simulink model "Rail_SetPoint"  (R2016b)
settings: configuration reference "CodeGenConfigSet" (kept outside this file)
values from neighbouring files (symbols this model uses):
  Rail_dpSetPointDec_CUR = Calibration.Parameter    [init_Rail_SetPoint.m]    (also in init_Rail_SetPoint_SIL.m = Simulink.Parameter)
  Rail_dpSetPointDec_CURX = Calibration.Parameter    [init_Rail_SetPoint.m]    (also in init_Rail_SetPoint_SIL.m = Simulink.Parameter)
  Rail_dpSetPointDec_MAP = Calibration.Parameter    [init_Rail_SetPoint.m]    (also in init_Rail_SetPoint_SIL.m = Simulink.Parameter)
  Rail_dpSetPointDec_MAPX = Calibration.Parameter    [init_Rail_SetPoint.m]    (also in init_Rail_SetPoint_SIL.m = Simulink.Parameter)
  Rail_dpSetPointDec_MAPY = Calibration.Parameter    [init_Rail_SetPoint.m]    (also in init_Rail_SetPoint_SIL.m = Simulink.Parameter)
  Rail_dpSetPointInc_MAP = Calibration.Parameter    [init_Rail_SetPoint.m]    (also in init_Rail_SetPoint_SIL.m = Simulink.Parameter)
  Rail_dpSetPointInc_MAPX = Calibration.Parameter    [init_Rail_SetPoint.m]    (also in init_Rail_SetPoint_SIL.m = Simulink.Parameter)
  Rail_dpSetPointInc_MAPY = Calibration.Parameter    [init_Rail_SetPoint.m]    (also in init_Rail_SetPoint_SIL.m = Simulink.Parameter)
  Rail_dpSetPointIncLim_MAP = Calibration.Parameter    [init_Rail_SetPoint.m]    (also in init_Rail_SetPoint_SIL.m = Simulink.Parameter)
  Rail_dpSetPointIncLim_MAPX = Calibration.Parameter    [init_Rail_SetPoint.m]    (also in init_Rail_SetPoint_SIL.m = Simulink.Parameter)
  Rail_dpSetPointIncLim_MAPY = Calibration.Parameter    [init_Rail_SetPoint.m]    (also in init_Rail_SetPoint_SIL.m = Simulink.Parameter)
  Rail_pEnvpSetPointIncHi_C = Calibration.Parameter    [init_Rail_SetPoint.m]    (also in init_Rail_SetPoint_SIL.m = Simulink.Parameter)
  Rail_pEnvpSetPointIncLo_C = Calibration.Parameter    [init_Rail_SetPoint.m]    (also in init_Rail_SetPoint_SIL.m = Simulink.Parameter)
  Rail_pSetPointBasEOM0_MAP = Calibration.Parameter    [init_Rail_SetPoint.m]    (also in init_Rail_SetPoint_SIL.m = Simulink.Parameter)
  Rail_pSetPointBasEOM0_MAPX = Calibration.Parameter    [init_Rail_SetPoint.m]    (also in init_Rail_SetPoint_SIL.m = Simulink.Parameter)
  Rail_pSetPointBasEOM0_MAPY = Calibration.Parameter    [init_Rail_SetPoint.m]    (also in init_Rail_SetPoint_SIL.m = Simulink.Parameter)
  Rail_pSetPointErrLoLim_CUR = Calibration.Parameter    [init_Rail_SetPoint.m]    (also in init_Rail_SetPoint_SIL.m = Simulink.Parameter)
  Rail_pSetPointErrLoLim_CURX = Calibration.Parameter    [init_Rail_SetPoint.m]    (also in init_Rail_SetPoint_SIL.m = Simulink.Parameter)
  Rail_pSetPointLimNFlTemp_MAP = Calibration.Parameter    [init_Rail_SetPoint.m]    (also in init_Rail_SetPoint_SIL.m = Simulink.Parameter)
  Rail_pSetPointLimNFlTemp_MAPX = Calibration.Parameter    [init_Rail_SetPoint.m]    (also in init_Rail_SetPoint_SIL.m = Simulink.Parameter)
  Rail_pSetPointLimNFlTemp_MAPY = Calibration.Parameter    [init_Rail_SetPoint.m]    (also in init_Rail_SetPoint_SIL.m = Simulink.Parameter)
  Rail_pSetPointRed_C = Calibration.Parameter    [init_Rail_SetPoint.m]    (also in init_Rail_SetPoint_SIL.m = Simulink.Parameter)
  Rail_swtDynLim_C = Calibration.Parameter    [init_Rail_SetPoint.m]    (also in init_Rail_SetPoint_SIL.m = Simulink.Parameter)
  Rail_swtIncLim_C = Calibration.Parameter    [init_Rail_SetPoint.m]    (also in init_Rail_SetPoint_SIL.m = Simulink.Parameter)
  Rail_swtPSetPointSrc_C = Calibration.Parameter    [init_Rail_SetPoint.m]    (also in init_Rail_SetPoint_SIL.m = Simulink.Parameter)
  Rail_swtqIncSel_C = Calibration.Parameter    [init_Rail_SetPoint.m]    (also in init_Rail_SetPoint_SIL.m = Simulink.Parameter)
  Rail_swtStatLim_C = Calibration.Parameter    [init_Rail_SetPoint.m]    (also in init_Rail_SetPoint_SIL.m = Simulink.Parameter)
  SigTst_pSetPoint_C = Calibration.Parameter    [init_Rail_SetPoint.m]    (also in init_Rail_SetPoint_SIL.m = Simulink.Parameter)
  SigTst_swtSetPoint_C = Calibration.Parameter    [init_Rail_SetPoint.m]    (also in init_Rail_SetPoint_SIL.m = Simulink.Parameter)
undefined symbols (not defined in the file or in its folder): EngState_conv, Rail_SetPoint_DT, RailCtl_State_conv, Switch_conv
libraries: CXLib x5
settings Model: Creator=lenovo  LastModifiedBy=dulinggang
settings ConfigSetRef: SourceLocation=Base Workspace

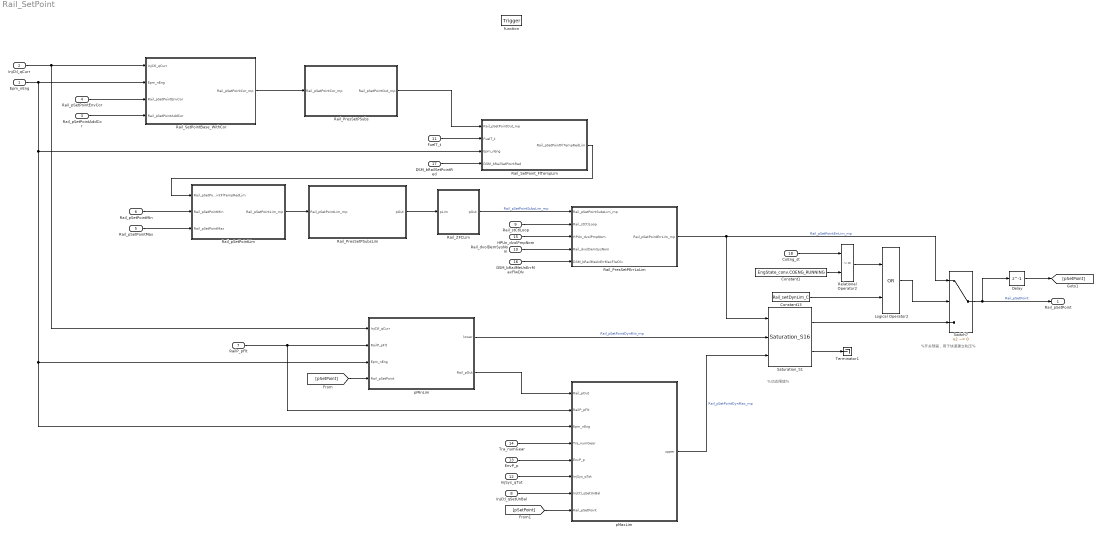
== system Rail_SetPoint ==
  note: %动态限值%
  note: %开关预留，用于快速建立轨压%
  Epm_nEng : Inport  Tag=rpm  Description=Engine speed  OutMin=0  OutMax=6000  OutDataTypeStr=EngSpeed_rpm
  InjCtl_qCurr : Inport  Tag=mg/hub  Description=Torque generating engine fuel injection quantity  Port=2  OutMin=-319  OutMax=319  OutDataTypeStr=FuelMass_mg_hub
  Rail_pSetPointAddCor : Inport  Tag=bar  Description=Buffer variable for additional correction rail setpoint values which were received via the remote function Rail_SetPointAddCor.  Port=3  OutMin=-2500  OutMax=2500  OutDataTypeStr=RailPressure_bar
  Rail_pSetPointEnvCor : Inport  Tag=bar  Description=Corrected rail pressure setpoint based on environmental conditions (for present operation mode)  Port=4  OutMin=-2500  OutMax=2500  OutDataTypeStr=RailPressure_bar
  Rail_pSetPointMax : Inport  Tag=bar  Description=Maximum rail pressure setpoint  Port=5  OutMin=-2500  OutMax=2500  OutDataTypeStr=RailPressure_bar
  Rail_pSetPointMin : Inport  Tag=bar  Description=Minimum rail pressure setpoint  Port=6  OutMin=-2500  OutMax=2500  OutDataTypeStr=RailPressure_bar
  RailP_pFlt : Inport  Tag=bar  Description=Maximum rail pressure of the last 10 sampling cycle  Port=7  OutMin=0  OutMax=2500  OutDataTypeStr=RailPressure_bar
  InjCtl_qSetUnBal : Inport  Tag=mg/hub  Description=Current injection quantity  Port=8  OutMin=-319  OutMax=319  OutDataTypeStr=FuelMass_mg_hub
  Rail_stCtlLoop : Inport  Description=State of the rail pressure governor control  Port=9  OutDataTypeStr=Enum: RailCtl_State_conv
  Rail_dvolDemSysNom : Inport  Tag=mm^3/s  Description=Volume flow demanded overall for a nominal injection system  Port=10  OutMin=-327680  OutMax=327670  OutDataTypeStr=FuelVol_mm3_s
  FuelT_t : Inport  Tag=deg  Description=Temperature of fuel  Port=11  OutMin=-50  OutMax=150  OutDataTypeStr=Temp_deg
  InjSys_qTot : Inport  Tag=mg/hub  Description=Total engine injection quantity  Port=12  OutMin=-319  OutMax=319  OutDataTypeStr=FuelMass_mg_hub
  EnvP_p : Inport  Tag=kPa  Description=Barometric pressure  Port=13  OutMin=0  OutMax=3276  OutDataTypeStr=AirPressure_kPa
  Tra_numGear : Inport  Description=Current gear information  Port=14  OutMin=-128  OutMax=127  OutDataTypeStr=Tra_num
  HPUn_dvolPmpNom : Inport  Tag=mm^3/s  Description=Pump Nominal value  Port=15  OutMin=0  OutMax=50000  OutDataTypeStr=FuelVol_mm3_s
  DSM_bRailMeUnErrMaxFlwDlv : Inport  Description=state of Fid_RailMeUnErrMaxFlwDlv  Port=16  OutMin=0  OutMax=1  OutDataTypeStr=boolean
  DSM_bRailSetPointRed : Inport  Description=state of FId_RailSetPointRed  Port=17  OutMin=0  OutMax=1  OutDataTypeStr=boolean
  CoEng_st : Inport  Description=Engine coordinator state  Port=18  OutDataTypeStr=Enum: EngState_conv
  function : TriggerPort  TriggerType=function-call  VariantControl=Variant
  Constant1 : Constant  Value=EngState_conv.COENG_RUNNING
  Constant13 : Constant  Value=Rail_swtDynLim_C
  Delay : Delay  DelayLength=1  InitialCondition=0
  Logical Operator2 : Logic  Operator=OR  AllPortsSameDT=off  OutDataTypeStr=boolean
  Rail_PresSetPErrLoLim : Subsystem
  Rail_PresSetPSubs : Subsystem
  Rail_PresSetPSubsLim : Subsystem
  Rail_SetPointBase_WithCor : Subsystem
  Rail_SetPoint_FlTempLim : Subsystem
  Rail_ZFCLim : Subsystem
  Rail_pSetPointLim : Subsystem
  Relational Operator2 : RelationalOperator  Operator=~=  OutDataTypeStr=boolean  RndMeth=Simplest  InputSameDT=on
  Saturation_S1 : CXLib/Saturation_S16  RequirementInfo={'other' 'Rail_requirements.doc' '@Simulink_requirement_item_42' 'true' '目标轨压动态限值' '' } %GIDa_002271f1_d5a1_4f79_991c_8acc6585766a
  Switch7 : Switch  Criteria=u2 ~= 0  InputSameDT=on
  Terminator1 : Terminator
  pMaxLim : Subsystem
  pMinLim : Subsystem
  Rail_pSetPoint : Outport  Tag=bar  Description=Rail pressure setpoint  OutMin=-2500  OutMax=2500  OutDataTypeStr=RailPressure_bar
  wires:
  Saturation_S1/1 -> Switch7/3
  Rail_SetPointBase_WithCor/1(Rail_pSetPointCor_mp) -> Rail_PresSetPSubs/1(Rail_pSetPointCor_mp)
  Rail_stCtlLoop/1 -> Rail_PresSetPErrLoLim/2(Rail_stCtlLoop)
  Rail_dvolDemSysNom/1 -> Rail_PresSetPErrLoLim/4(Rail_dvolDemSysNom)
  HPUn_dvolPmpNom/1 -> Rail_PresSetPErrLoLim/3(HPUn_dvolPmpNom)
  Delay/1 -> [pSetPoint]
  Switch7/1 -> Rail_pSetPoint/1, Delay/1  "Rail_pSetPoint"
  RailP_pFlt/1 -> pMinLim/2(RailP_pFlt), pMaxLim/2(RailP_pFlt)
  Saturation_S1/2 -> Terminator1/1
  Rail_PresSetPErrLoLim/1(Rail_pSetPointErrLim_mp) -> Switch7/1, Saturation_S1/1  "Rail_pSetPointErrLim_mp"
  Rail_ZFCLim/1(pOut) -> Rail_PresSetPErrLoLim/1(Rail_pSetPointSubsLim_mp)  "Rail_pSetPointSubsLim_mp"
  Rail_PresSetPSubsLim/1(pOut) -> Rail_ZFCLim/1(pLim)
  Rail_pSetPointEnvCor/1 -> Rail_SetPointBase_WithCor/3(Rail_pSetPointEnvCor)
  Rail_pSetPointAddCor/1 -> Rail_SetPointBase_WithCor/4(Rail_pSetPointAddCor)
  Epm_nEng/1 -> pMaxLim/3(Epm_nEng), pMinLim/3(Epm_nEng), Rail_SetPoint_FlTempLim/3(Epm_nEng), Rail_SetPointBase_WithCor/2(Epm_nEng)
  InjCtl_qCurr/1 -> pMinLim/1(InjCtl_qCurr), Rail_SetPointBase_WithCor/1(InjCtl_qCurr)
  DSM_bRailMeUnErrMaxFlwDlv/1 -> Rail_PresSetPErrLoLim/5(DSM_bRailMeUnErrMaxFlwDlv)
  Rail_PresSetPSubs/1(Rail_pSetPointOut_mp) -> Rail_SetPoint_FlTempLim/1(Rail_pSetPointOut_mp)
  FuelT_t/1 -> Rail_SetPoint_FlTempLim/2(FuelT_t)
  DSM_bRailSetPointRed/1 -> Rail_SetPoint_FlTempLim/4(DSM_bRailSetPointRed)
  Rail_SetPoint_FlTempLim/1(Rail_pSetPointFlTempRedLim) -> Rail_pSetPointLim/1(Rail_pSetPointFlTempRedLim)
  Rail_pSetPointMin/1 -> Rail_pSetPointLim/2(Rail_pSetPointMin)
  Rail_pSetPointMax/1 -> Rail_pSetPointLim/3(Rail_pSetPointMax)
  Rail_pSetPointLim/1(Rail_pSetPointLim_mp) -> Rail_PresSetPSubsLim/1(Rail_pSetPointLim_mp)
  pMinLim/1(lower) -> Saturation_S1/2  "Rail_pSetPointDynMin_mp"
  pMinLim/2(Rail_pOut) -> pMaxLim/1(Rail_pOut)
  Tra_numGear/1 -> pMaxLim/4(Tra_numGear)
  EnvP_p/1 -> pMaxLim/5(EnvP_p)
  InjSys_qTot/1 -> pMaxLim/6(InjSys_qTot)
  InjCtl_qSetUnBal/1 -> pMaxLim/7(InjCtl_qSetUnBal)
  pMaxLim/1(upper) -> Saturation_S1/3  "Rail_pSetPointDynMax_mp"
  [pSetPoint] -> pMinLim/4(Rail_pSetPoint)
  [pSetPoint] -> pMaxLim/8(Rail_pSetPoint)
  CoEng_st/1 -> Relational Operator2/1
  Constant1/1 -> Relational Operator2/2
  Relational Operator2/1 -> Logical Operator2/1
  Constant13/1 -> Logical Operator2/2
  Logical Operator2/1 -> Switch7/2

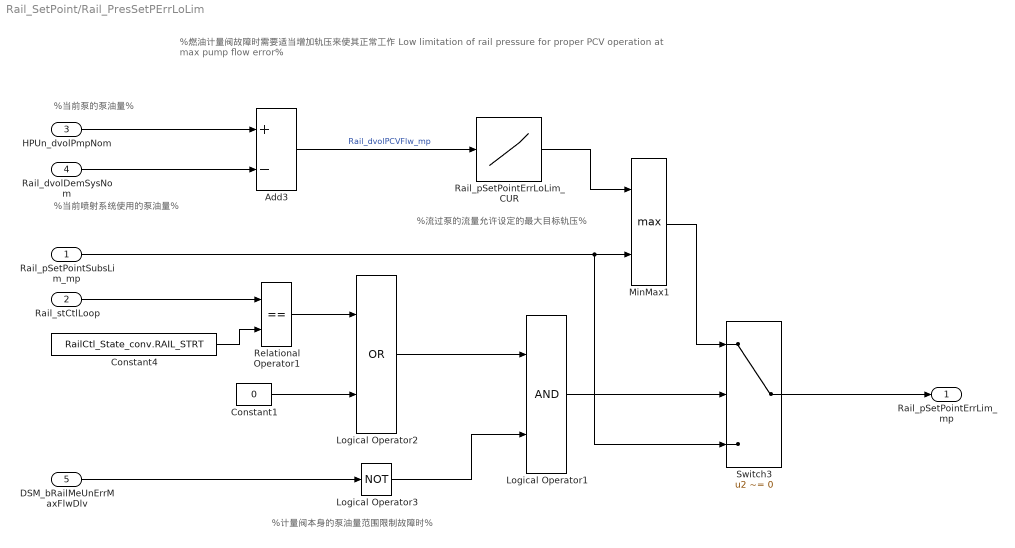
== system Rail_SetPoint/Rail_PresSetPErrLoLim ==
  note: %燃油计量阀故障时需要适当增加轨压来使其正常工作
      | Low limitation of rail pressure for proper PCV operation at max pump ﬂow error%
  note: %当前泵的泵油量%
  note: %当前喷射系统使用的泵油量%
  note: %流过泵的流量允许设定的最大目标轨压%
  note: %计量阀本身的泵油量范围限制故障时%
  Rail_pSetPointSubsLim_mp : Inport
  Rail_stCtlLoop : Inport  Port=2
  HPUn_dvolPmpNom : Inport  Port=3
  Rail_dvolDemSysNom : Inport  Port=4
  DSM_bRailMeUnErrMaxFlwDlv : Inport  Description=state of Fid_RailMeUnErrMaxFlwDlv  Port=5  OutMin=0  OutMax=1  OutDataTypeStr=boolean
  Add3 : Sum  Inputs=+-  OutDataTypeStr=Inherit: Inherit via back propagation  InputSameDT=on
  Constant1 : Constant  Value=0  OutDataTypeStr=Inherit: Inherit via back propagation
  Constant4 : Constant  Value=RailCtl_State_conv.RAIL_STRT
  Logical Operator1 : Logic  AllPortsSameDT=off  OutDataTypeStr=boolean
  Logical Operator2 : Logic  Operator=OR  AllPortsSameDT=off  OutDataTypeStr=boolean
  Logical Operator3 : Logic  Operator=NOT  AllPortsSameDT=off  OutDataTypeStr=boolean
  MinMax1 : MinMax  Function=max  Inputs=2  InputSameDT=on
  Rail_pSetPointErrLoLim_CUR : Lookup_n-D  NumberOfTableDimensions=1  BreakpointsForDimension1=Rail_pSetPointErrLoLim_CURX  BreakpointsForDimension2=Rail_dpSetPointDec_MAPX  IndexSearchMethod=Linear search  Table=Rail_pSetPointErrLoLim_CUR  ExtrapMethod=Clip  InternalRulePriority=Speed  OutDataTypeStr=Inherit: Inherit via back propagation  RndMeth=Simplest  SaturateOnIntegerOverflow=on
  Relational Operator1 : RelationalOperator  Operator===  OutDataTypeStr=boolean  RndMeth=Nearest  InputSameDT=on
  Switch3 : Switch  Criteria=u2 ~= 0  InputSameDT=on
  Rail_pSetPointErrLim_mp : Outport
  wires:
  Logical Operator3/1 -> Logical Operator1/2
  Rail_dvolDemSysNom/1 -> Add3/2
  Switch3/1 -> Rail_pSetPointErrLim_mp/1
  MinMax1/1 -> Switch3/1
  Add3/1 -> Rail_pSetPointErrLoLim_CUR/1  "Rail_dvolPCVFlw_mp"
  Rail_pSetPointErrLoLim_CUR/1 -> MinMax1/1
  Rail_pSetPointSubsLim_mp/1 -> MinMax1/2, Switch3/3
  DSM_bRailMeUnErrMaxFlwDlv/1 -> Logical Operator3/1
  Logical Operator2/1 -> Logical Operator1/1
  Constant4/1 -> Relational Operator1/2
  Constant1/1 -> Logical Operator2/2
  Relational Operator1/1 -> Logical Operator2/1
  Logical Operator1/1 -> Switch3/2
  Rail_stCtlLoop/1 -> Relational Operator1/1
  HPUn_dvolPmpNom/1 -> Add3/1

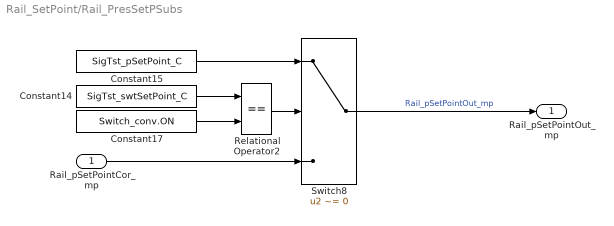
== system Rail_SetPoint/Rail_PresSetPSubs ==
  Rail_pSetPointCor_mp : Inport
  Constant14 : Constant  Value=SigTst_swtSetPoint_C
  Constant15 : Constant  Value=SigTst_pSetPoint_C
  Constant17 : Constant  RequirementInfo={'other' 'APP_requirements.doc' '@Simulink_requirement_item_25' 'true' '手动开关' '' } %GIDa_ecdab07e_4532_49c0_ab83_fe11a5eac9af  Value=Switch_conv.ON  OutDataTypeStr=Inherit: Inherit via back propagation
  Relational Operator2 : RelationalOperator  Operator===  OutDataTypeStr=boolean  RndMeth=Simplest  InputSameDT=on
  Switch8 : Switch  Criteria=u2 ~= 0  InputSameDT=on
  Rail_pSetPointOut_mp : Outport
  wires:
  Switch8/1 -> Rail_pSetPointOut_mp/1  "Rail_pSetPointOut_mp"
  Constant17/1 -> Relational Operator2/2
  Relational Operator2/1 -> Switch8/2
  Constant15/1 -> Switch8/1
  Constant14/1 -> Relational Operator2/1
  Rail_pSetPointCor_mp/1 -> Switch8/3

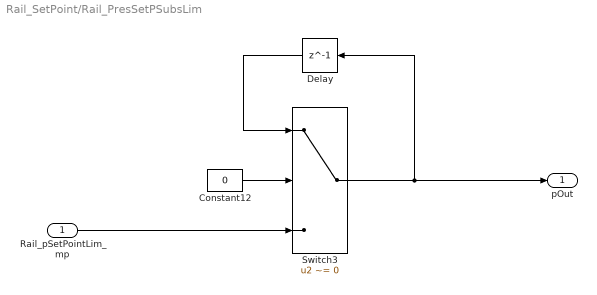
== system Rail_SetPoint/Rail_PresSetPSubsLim ==
  Rail_pSetPointLim_mp : Inport
  Constant12 : Constant  Value=0  OutDataTypeStr=boolean
  Delay : Delay  DelayLength=1  InitialCondition=0
  Switch3 : Switch  Criteria=u2 ~= 0
  pOut : Outport
  wires:
  Delay/1 -> Switch3/1
  Constant12/1 -> Switch3/2
  Switch3/1 -> pOut/1, Delay/1
  Rail_pSetPointLim_mp/1 -> Switch3/3

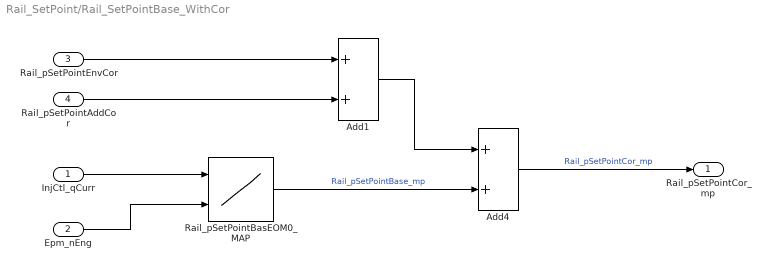
== system Rail_SetPoint/Rail_SetPointBase_WithCor ==
  InjCtl_qCurr : Inport
  Epm_nEng : Inport  Port=2
  Rail_pSetPointEnvCor : Inport  Port=3
  Rail_pSetPointAddCor : Inport  Port=4
  Add1 : Sum  RequirementInfo={'other' 'Rail_requirements.doc' '@Simulink_requirement_item_35' 'true' '基础目标轨压计算' '' } %GIDa_3374ff71_837a_4a3b_b639_fcdda33b3c53  InputSameDT=on
  Add4 : Sum  RequirementInfo={'other' 'Rail_requirements.doc' '@Simulink_requirement_item_35' 'true' '基础目标轨压计算' '' } %GIDa_9e013fe7_9a80_4710_931c_50a6c6a28086  InputSameDT=on
  Rail_pSetPointBasEOM0_MAP : Lookup_n-D  RequirementInfo={'other' 'Rail_requirements.doc' '@Simulink_requirement_item_35' 'true' '基础目标轨压计算' '' } %GIDa_e29dad87_2f5f_485f_b5b2_04a6cc9fd0a8  BreakpointsForDimension1=Rail_pSetPointBasEOM0_MAPY  BreakpointsForDimension2=Rail_pSetPointBasEOM0_MAPX  BreakpointsForDimension1DataTypeStr=Inherit: Inherit from 'Breakpoint data'  BreakpointsForDimension2DataTypeStr=Inherit: Inherit from 'Breakpoint data'  IndexSearchMethod=Linear search  Table=Rail_pSetPointBasEOM0_MAP  ExtrapMethod=Clip  InternalRulePriority=Speed  OutDataTypeStr=Inherit: Inherit via back propagation  RndMeth=Simplest  SaturateOnIntegerOverflow=on
  Rail_pSetPointCor_mp : Outport
  wires:
  Add4/1 -> Rail_pSetPointCor_mp/1  "Rail_pSetPointCor_mp"
  Add1/1 -> Add4/1
  Rail_pSetPointAddCor/1 -> Add1/2
  Rail_pSetPointEnvCor/1 -> Add1/1
  Rail_pSetPointBasEOM0_MAP/1 -> Add4/2  "Rail_pSetPointBase_mp"
  Epm_nEng/1 -> Rail_pSetPointBasEOM0_MAP/2
  InjCtl_qCurr/1 -> Rail_pSetPointBasEOM0_MAP/1

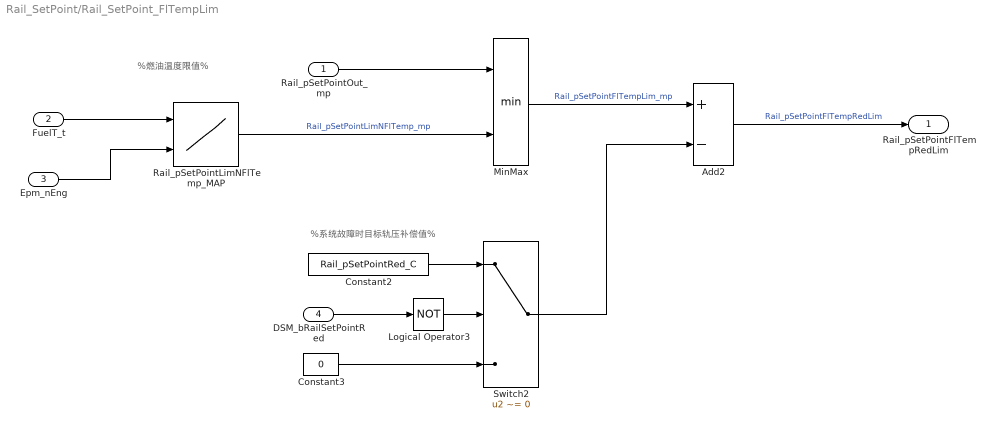
== system Rail_SetPoint/Rail_SetPoint_FlTempLim ==
  note: %燃油温度限值%
  note: %系统故障时目标轨压补偿值%
  Rail_pSetPointOut_mp : Inport
  FuelT_t : Inport  Tag=deg  Description=Temperature of fuel  Port=2  OutMin=-50  OutMax=200  OutDataTypeStr=Temp_deg
  Epm_nEng : Inport  Port=3
  DSM_bRailSetPointRed : Inport  Description=state of FId_RailSetPointRed  Port=4  OutMin=0  OutMax=1  OutDataTypeStr=boolean
  Add2 : Sum  Inputs=+-  OutDataTypeStr=Inherit: Inherit via back propagation  InputSameDT=on
  Constant2 : Constant  Value=Rail_pSetPointRed_C
  Constant3 : Constant  Value=0  OutDataTypeStr=Inherit: Inherit via back propagation
  Logical Operator3 : Logic  Operator=NOT  AllPortsSameDT=off  OutDataTypeStr=boolean
  MinMax : MinMax  Inputs=2  InputSameDT=on
  Rail_pSetPointLimNFlTemp_MAP : Lookup_n-D  RequirementInfo={'other' 'Rail_requirements.doc' '@Simulink_requirement_item_37' 'true' '燃油温度限值计算' '' } %GIDa_aa5a5aa3_0e0e_41b4_9ff8_04ca51c73c82  BreakpointsForDimension1=Rail_pSetPointLimNFlTemp_MAPY  BreakpointsForDimension2=Rail_pSetPointLimNFlTemp_MAPX  BreakpointsForDimension1DataTypeStr=Inherit: Inherit from 'Breakpoint data'  BreakpointsForDimension2DataTypeStr=Inherit: Inherit from 'Breakpoint data'  IndexSearchMethod=Linear search  Table=Rail_pSetPointLimNFlTemp_MAP  ExtrapMethod=Clip  InternalRulePriority=Speed  OutDataTypeStr=Inherit: Inherit via back propagation  RndMeth=Simplest  SaturateOnIntegerOverflow=on
  Switch2 : Switch  Criteria=u2 ~= 0  InputSameDT=on
  Rail_pSetPointFlTempRedLim : Outport
  wires:
  Logical Operator3/1 -> Switch2/2
  Add2/1 -> Rail_pSetPointFlTempRedLim/1  "Rail_pSetPointFlTempRedLim"
  Switch2/1 -> Add2/2
  Constant3/1 -> Switch2/3
  Constant2/1 -> Switch2/1
  DSM_bRailSetPointRed/1 -> Logical Operator3/1
  MinMax/1 -> Add2/1  "Rail_pSetPointFlTempLim_mp"
  Rail_pSetPointLimNFlTemp_MAP/1 -> MinMax/2  "Rail_pSetPointLimNFlTemp_mp"
  FuelT_t/1 -> Rail_pSetPointLimNFlTemp_MAP/1
  Rail_pSetPointOut_mp/1 -> MinMax/1
  Epm_nEng/1 -> Rail_pSetPointLimNFlTemp_MAP/2

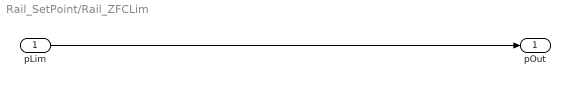
== system Rail_SetPoint/Rail_ZFCLim ==
  pLim : Inport
  pOut : Outport
  wires:
  pLim/1 -> pOut/1

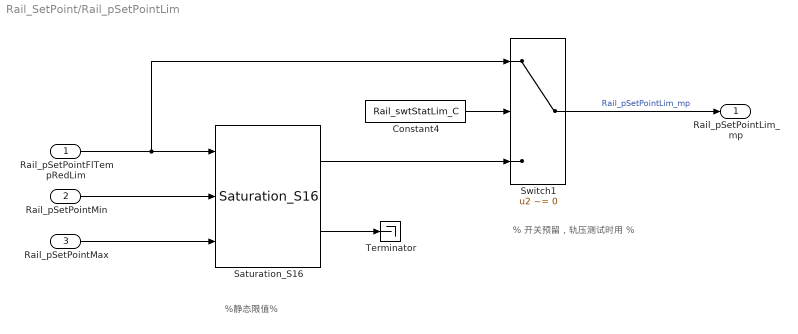
== system Rail_SetPoint/Rail_pSetPointLim ==
  note: %静态限值%
  note: % 开关预留，轨压测试时用 %
  Rail_pSetPointFlTempRedLim : Inport
  Rail_pSetPointMin : Inport  Tag=bar  Description=Minimum rail pressure setpoint  Port=2  OutMin=0  OutMax=2500  OutDataTypeStr=RailPressure_bar
  Rail_pSetPointMax : Inport  Tag=bar  Description=Maximum rail pressure setpoint  Port=3  OutMin=0  OutMax=2500  OutDataTypeStr=RailPressure_bar
  Constant4 : Constant  Value=Rail_swtStatLim_C
  Saturation_S16 : CXLib/Saturation_S16  RequirementInfo={'other' 'Rail_requirements.doc' '@Simulink_requirement_item_38' 'true' '目标轨压静态限制' '' } %GIDa_8529386c_3cc7_4201_b8d8_d01e3fb27ed5
  Switch1 : Switch  Criteria=u2 ~= 0  SaturateOnIntegerOverflow=on  InputSameDT=on
  Terminator : Terminator
  Rail_pSetPointLim_mp : Outport
  wires:
  Saturation_S16/1 -> Switch1/3
  Switch1/1 -> Rail_pSetPointLim_mp/1  "Rail_pSetPointLim_mp"
  Constant4/1 -> Switch1/2
  Saturation_S16/2 -> Terminator/1
  Rail_pSetPointMin/1 -> Saturation_S16/2
  Rail_pSetPointMax/1 -> Saturation_S16/3
  Rail_pSetPointFlTempRedLim/1 -> Switch1/1, Saturation_S16/1

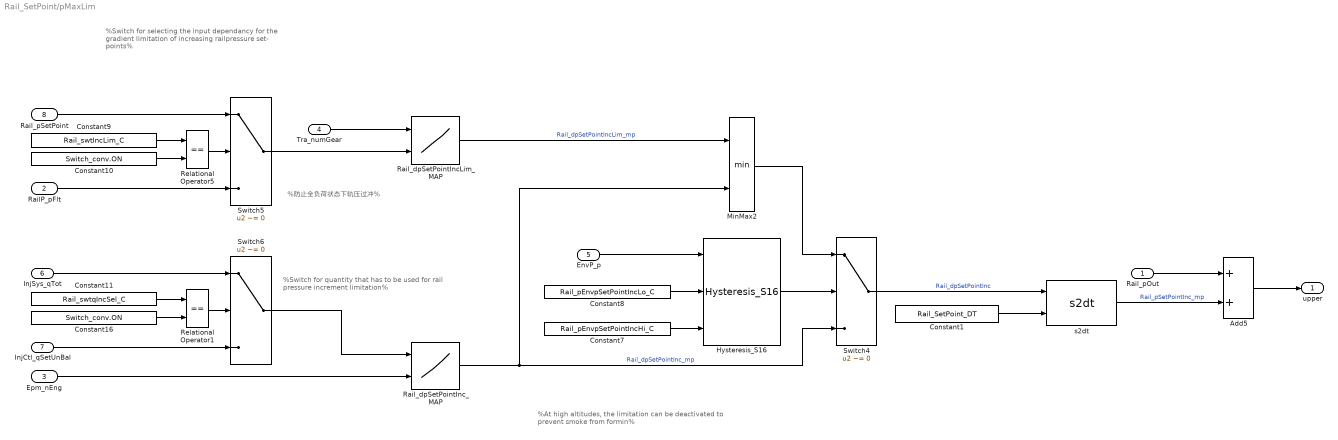
== system Rail_SetPoint/pMaxLim ==
  note: %At high altitudes, the limitation can be deactivated
      | to prevent smoke from formin%
  note: %Switch for selecting the input dependancy for the
      | gradient limitation of increasing railpressure set-
      | points%
  note: %Switch for quantity that has to be used for rail
      | pressure increment limitation%
  note: %防止全负荷状态下轨压过冲%
  Rail_pOut : Inport
  RailP_pFlt : Inport  Port=2
  Epm_nEng : Inport  Port=3
  Tra_numGear : Inport  Description=Current gear information  Port=4  OutMin=-128  OutMax=127  OutDataTypeStr=Tra_num
  EnvP_p : Inport  Tag=kPa  Description=atmospheric pressure actual physical value  Port=5  OutMin=0  OutMax=350  OutDataTypeStr=AirPressure_kPa
  InjSys_qTot : Inport  Tag=mg/hub  Description=Total engine injection quantity  Port=6  OutMin=0  OutMax=300  OutDataTypeStr=FuelMass_mg_hub
  InjCtl_qSetUnBal : Inport  Tag=mg/hub  Description=current injection quantity  Port=7  OutMin=0  OutMax=300  OutDataTypeStr=FuelMass_mg_hub
  Rail_pSetPoint : Inport  Port=8
  Add5 : Sum  RequirementInfo={'other' 'Rail_requirements.doc' '@Simulink_requirement_item_41' 'true' '动态增加模块' '' } %GIDa_bcf758d9_44e9_4c32_84c7_4b8421d5894c  InputSameDT=on
  Constant1 : Constant  Value=Rail_SetPoint_DT
  Constant10 : Constant  RequirementInfo={'other' 'APP_requirements.doc' '@Simulink_requirement_item_25' 'true' '手动开关' '' } %GIDa_525d88b8_b1df_4b5e_859a_1e3fdc551e01  Value=Switch_conv.ON  OutDataTypeStr=Inherit: Inherit via back propagation
  Constant11 : Constant  RequirementInfo={'other' 'Rail_requirements.doc' '@Simulink_requirement_item_41' 'true' '动态增加模块' '' } %GIDa_0d31823b_075e_4d39_8d1e_828fe3f3d2a8  Value=Rail_swtqIncSel_C
  Constant16 : Constant  RequirementInfo={'other' 'APP_requirements.doc' '@Simulink_requirement_item_25' 'true' '手动开关' '' } %GIDa_9fd35118_2ad0_4c76_bead_6d3f9a27e3b7  Value=Switch_conv.ON  OutDataTypeStr=Inherit: Inherit via back propagation
  Constant7 : Constant  RequirementInfo={'other' 'Rail_requirements.doc' '@Simulink_requirement_item_41' 'true' '动态增加模块' '' } %GIDa_7e671a68_ab3e_4d02_add3_840afbbc8d84  Value=Rail_pEnvpSetPointIncHi_C
  Constant8 : Constant  RequirementInfo={'other' 'Rail_requirements.doc' '@Simulink_requirement_item_41' 'true' '动态增加模块' '' } %GIDa_7ae424bd_506c_4b51_878a_3f1376c79fff  Value=Rail_pEnvpSetPointIncLo_C
  Constant9 : Constant  RequirementInfo={'other' 'Rail_requirements.doc' '@Simulink_requirement_item_41' 'true' '动态增加模块' '' } %GIDa_d249bd79_e106_4950_ba0b_9546d15d2ad7  Value=Rail_swtIncLim_C
  Hysteresis_S16 : CXLib/Hysteresis_S16  RequirementInfo={'other' 'Rail_requirements.doc' '@Simulink_requirement_item_41' 'true' '动态增加模块' '' } %GIDa_3452b730_920e_47b0_aa1a_90ade8fdfafd
  MinMax2 : MinMax  RequirementInfo={'other' 'Rail_requirements.doc' '@Simulink_requirement_item_41' 'true' '动态增加模块' '' } %GIDa_f8e94196_e856_4634_a61b_43e499696b08  Inputs=2  InputSameDT=on
  Rail_dpSetPointIncLim_MAP : Lookup_n-D  RequirementInfo={'other' 'Rail_requirements.doc' '@Simulink_requirement_item_41' 'true' '动态增加模块' '' } %GIDa_2a861fba_5c02_4eed_9f83_48b894cd0268  BreakpointsForDimension1=Rail_dpSetPointIncLim_MAPY  BreakpointsForDimension2=Rail_dpSetPointIncLim_MAPX  BreakpointsForDimension1DataTypeStr=Inherit: Inherit from 'Breakpoint data'  BreakpointsForDimension2DataTypeStr=Inherit: Inherit from 'Breakpoint data'  IndexSearchMethod=Linear search  Table=Rail_dpSetPointIncLim_MAP  ExtrapMethod=Clip  InternalRulePriority=Speed  OutDataTypeStr=Inherit: Inherit via back propagation  RndMeth=Simplest  SaturateOnIntegerOverflow=on
  Rail_dpSetPointInc_MAP : Lookup_n-D  RequirementInfo={'other' 'Rail_requirements.doc' '@Simulink_requirement_item_41' 'true' '动态增加模块' '' } %GIDa_604ad5ff_c92b_4c9b_8fc9_5edb3f2e3e9f  BreakpointsForDimension1=Rail_dpSetPointInc_MAPY  BreakpointsForDimension2=Rail_dpSetPointInc_MAPX  BreakpointsForDimension1DataTypeStr=Inherit: Inherit from 'Breakpoint data'  BreakpointsForDimension2DataTypeStr=Inherit: Inherit from 'Breakpoint data'  IndexSearchMethod=Linear search  Table=Rail_dpSetPointInc_MAP  ExtrapMethod=Clip  InternalRulePriority=Speed  OutDataTypeStr=Inherit: Inherit via back propagation  RndMeth=Simplest  SaturateOnIntegerOverflow=on
  Relational Operator1 : RelationalOperator  Operator===  OutDataTypeStr=boolean  RndMeth=Simplest  InputSameDT=on
  Relational Operator5 : RelationalOperator  Operator===  OutDataTypeStr=boolean  RndMeth=Simplest  InputSameDT=on
  Switch4 : Switch  RequirementInfo={'other' 'Rail_requirements.doc' '@Simulink_requirement_item_41' 'true' '动态增加模块' '' } %GIDa_734c38b8_dfe2_49da_9c59_01b23b563dbe  Criteria=u2 ~= 0  InputSameDT=on
  Switch5 : Switch  RequirementInfo={'other' 'Rail_requirements.doc' '@Simulink_requirement_item_41' 'true' '动态增加模块' '' } %GIDa_bab4e27e_ede4_4377_9c4d_fe7b98460f84  Criteria=u2 ~= 0  InputSameDT=on
  Switch6 : Switch  RequirementInfo={'other' 'Rail_requirements.doc' '@Simulink_requirement_item_41' 'true' '动态增加模块' '' } %GIDa_c38ca6d6_3369_4c28_b3a5_60da3530becd  Criteria=u2 ~= 0  InputSameDT=on
  s2dt : CXLib/s2dt
  upper : Outport
  wires:
  InjCtl_qSetUnBal/1 -> Switch6/3
  InjSys_qTot/1 -> Switch6/1
  Constant11/1 -> Relational Operator1/1
  Switch6/1 -> Rail_dpSetPointInc_MAP/1
  Add5/1 -> upper/1
  Rail_dpSetPointInc_MAP/1 -> MinMax2/2, Switch4/3  "Rail_dpSetPointInc_mp"
  Rail_pSetPoint/1 -> Switch5/1
  Constant9/1 -> Relational Operator5/1
  Switch5/1 -> Rail_dpSetPointIncLim_MAP/2
  Tra_numGear/1 -> Rail_dpSetPointIncLim_MAP/1
  Rail_dpSetPointIncLim_MAP/1 -> MinMax2/1  "Rail_dpSetPointIncLim_mp"
  Hysteresis_S16/1 -> Switch4/2
  Constant8/1 -> Hysteresis_S16/2
  Constant7/1 -> Hysteresis_S16/3
  EnvP_p/1 -> Hysteresis_S16/1
  MinMax2/1 -> Switch4/1
  Constant16/1 -> Relational Operator1/2
  Constant10/1 -> Relational Operator5/2
  Relational Operator1/1 -> Switch6/2
  Relational Operator5/1 -> Switch5/2
  s2dt/1 -> Add5/2  "Rail_pSetPointInc_mp"
  Switch4/1 -> s2dt/1  "Rail_dpSetPointInc"
  Rail_pOut/1 -> Add5/1
  RailP_pFlt/1 -> Switch5/3
  Epm_nEng/1 -> Rail_dpSetPointInc_MAP/2
  Constant1/1 -> s2dt/2

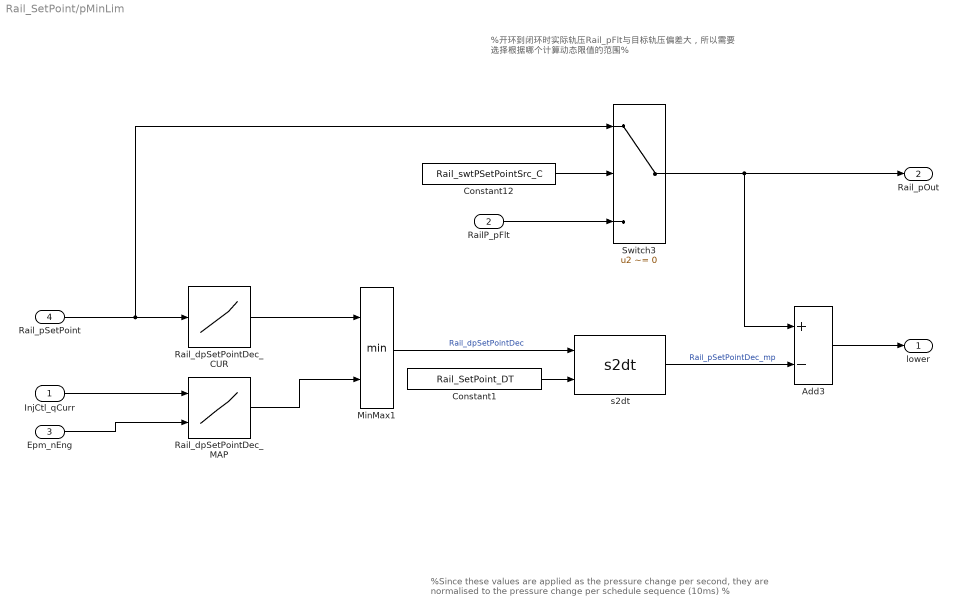
== system Rail_SetPoint/pMinLim ==
  note: %开环到闭环时实际轨压Rail_pFlt与目标轨压偏差大，所以需要
      | 选择根据哪个计算动态限值的范围%
  note: %Since these values are applied as the pressure change per second,
      | they are normalised to the pressure change per schedule sequence (10ms) %
  InjCtl_qCurr : Inport
  RailP_pFlt : Inport  Port=2
  Epm_nEng : Inport  Port=3
  Rail_pSetPoint : Inport  Port=4
  Add3 : Sum  RequirementInfo={'other' 'Rail_requirements.doc' '@Simulink_requirement_item_40' 'true' '动态减小模块' '' } %GIDa_01f6d098_112a_4de4_a2be_ed54ddb7e353  Inputs=+-  OutDataTypeStr=Inherit: Inherit via back propagation  InputSameDT=on
  Constant1 : Constant  Value=Rail_SetPoint_DT
  Constant12 : Constant  Value=Rail_swtPSetPointSrc_C
  MinMax1 : MinMax  RequirementInfo={'other' 'Rail_requirements.doc' '@Simulink_requirement_item_40' 'true' '动态减小模块' '' } %GIDa_b16fd65a_03cf_4ea1_8cc3_0a94811e7f01  Inputs=2  InputSameDT=on
  Rail_dpSetPointDec_CUR : Lookup_n-D  RequirementInfo={'other' 'Rail_requirements.doc' '@Simulink_requirement_item_40' 'true' '动态减小模块' '' } %GIDa_e32d72b6_915f_48b2_b4aa_f637fd2b6bdd  NumberOfTableDimensions=1  BreakpointsForDimension1=Rail_dpSetPointDec_CURX  BreakpointsForDimension2=Rail_dpSetPointDec_MAPX  IndexSearchMethod=Linear search  Table=Rail_dpSetPointDec_CUR  ExtrapMethod=Clip  InternalRulePriority=Speed  OutDataTypeStr=Inherit: Inherit via back propagation  RndMeth=Simplest  SaturateOnIntegerOverflow=on
  Rail_dpSetPointDec_MAP : Lookup_n-D  RequirementInfo={'other' 'Rail_requirements.doc' '@Simulink_requirement_item_40' 'true' '动态减小模块' '' } %GIDa_4abc1980_e658_40f6_b55f_19a0af7b177b  BreakpointsForDimension1=Rail_dpSetPointDec_MAPY  BreakpointsForDimension2=Rail_dpSetPointDec_MAPX  IndexSearchMethod=Linear search  Table=Rail_dpSetPointDec_MAP  ExtrapMethod=Clip  InternalRulePriority=Speed  OutDataTypeStr=Inherit: Inherit via back propagation  RndMeth=Simplest  SaturateOnIntegerOverflow=on
  Switch3 : Switch  RequirementInfo={'other' 'Rail_requirements.doc' '@Simulink_requirement_item_40' 'true' '动态减小模块' '' } %GIDa_fbff0e4d_51ca_4168_bd7f_20eaa331b42b  Criteria=u2 ~= 0  InputSameDT=on
  s2dt : CXLib/s2dt
  lower : Outport
  Rail_pOut : Outport  Port=2
  wires:
  Constant12/1 -> Switch3/2
  Rail_pSetPoint/1 -> Rail_dpSetPointDec_CUR/1, Switch3/1
  Add3/1 -> lower/1
  Switch3/1 -> Add3/1, Rail_pOut/1
  Rail_dpSetPointDec_MAP/1 -> MinMax1/2
  Rail_dpSetPointDec_CUR/1 -> MinMax1/1
  s2dt/1 -> Add3/2  "Rail_pSetPointDec_mp"
  MinMax1/1 -> s2dt/1  "Rail_dpSetPointDec"
  RailP_pFlt/1 -> Switch3/3
  Epm_nEng/1 -> Rail_dpSetPointDec_MAP/2
  InjCtl_qCurr/1 -> Rail_dpSetPointDec_MAP/1
  Constant1/1 -> s2dt/2
